simulink model "Diode"  (R2020b)
settings: Solver=VariableStepAuto  StartTime=0.0  StopTime=10.0  RelTol=1e-3
undefined symbols (not defined in the file): diodeCurrent, diodeVolts
settings Model: Creator=Shubham  LastModifiedBy=Shubham
settings DataIOCC: ExternalInput=[x, y]  SaveFormat=Array  ReturnWorkspaceOutputs=off  OutputSaveName=output

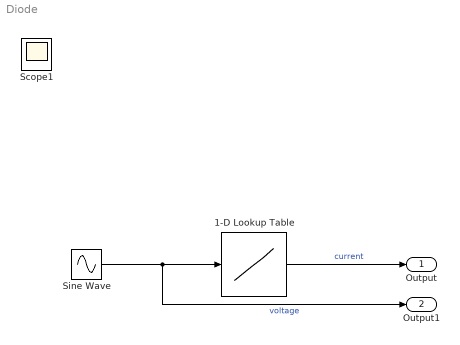
== system Diode ==
  1-D Lookup Table : Lookup_n-D  NumberOfTableDimensions=1  BreakpointsForDimension1=diodeVolts  Table=diodeCurrent  InternalRulePriority=Speed  RndMeth=Simplest  InputSameDT=on
  Sine Wave : Sin  Amplitude=0.5  Bias=1  SampleTime=0
  Output : Outport
  Output1 : Outport  Port=2
  Scope1 : Scope
  wires:
  Sine Wave/1 -> Output1/1, 1-D Lookup Table/1  "voltage"
  1-D Lookup Table/1 -> Output/1  "current"
